simulink model "dig_int_kurt"  (Simulink 6.2)
settings: Solver=ode45  StartTime=0.0  StopTime=1  RelTol=1e-3
undefined symbols (not defined in the file): bit_rev, iBOB, pfb_coeff_gen_calc
libraries: xbsIndex_r3 x1084, casper_library x95, xps_library x32
(part 2 of 8)

== system dig_int_kurt/cram1 ==
  In1 : Inport  Port=1  LatchInput=off
  In2 : Inport  Port=2  LatchInput=off
  In3 : Inport  Port=3  LatchInput=off
  In4 : Inport  Port=4  LatchInput=off
  In5 : Inport  Port=5  LatchInput=off
  In6 : Inport  Port=6  LatchInput=off
  Concat : S-Function  AncestorBlock=xbsIndex_r3/Concat  FunctionName=xlconcat  Parameters=sfcn_mwsv__  mask(Xilinx Bus Concatenator){num_inputs=6, explicit_period=off, period=1, dbl_ovrd=off}
      mask prompts: num_inputs "Number of Inputs"; explicit_period "Use Explicit Sample Period"; period "Sample Period  (use -1 to inherit first known input period)"; dbl_ovrd "Override with Doubles"
      mask help: Concatenates two or more inputs. Inputs must be unsigned with binary point at zero.
      mask init:
      | [designRoot, family, part, speed, package, simulinkPeriod, sysclkPeriod, dbl_ovrd, trimVbit] = xlSysgenSettings(gcb,1,1);
      | [bg,fg] = xlcmap('XBlock',dbl_ovrd);
      | iPos = get_param(gcb,'Position');
      | iWidth=iPos(3)-iPos(1); iHeight=iPos(4)-iPos(2);
      | iCx=iWidth/2;
      | iCy=iHeight/2;
      | [logoX, logoY] = xlogo(iPos);
      | 
      | 
      | 
      | 
      | % one time added for param list
      | numInputs = num_inputs + 1;
      | precision0 = 1;
      | latency = 0;
      | dblOvrd = dbl_ovrd;
      | explicitClk = explicit_period;
      | 
      | 
      | % just pass everything to s-function
      | sfcn_mwsv__ = get_param(gcb, 'MaskWSVariables');
      mask Help: eval('xlWeb(xlhtmldoclink(''Concat''))');
      mask StyleString: popup(2|3|4|5|6|7|8|9|10|11|12|13|14|15|16),checkbox,edit,checkbox
      mask CallbackString: |xlMagicCallback||
      mask Display:
      | patch([0 iWidth iWidth 0],[0 0 iHeight iHeight] , bg);
      | patch(logoX,logoY, fg);
      | port_label('input',1,'hi');
      | port_label('input',num_inputs+1,'lo');
      | port_label('output',1,'cat');
      | ;plot([0 0 iWidth iWidth 0], [0 iHeight iHeight 0 0]);
  Reinterp{1..6} (6 alike) : xbsIndex_r3/Reinterpret  force_arith_type=on  arith_type=Unsigned  force_bin_pt=on  bin_pt=0  force_valid=on
  Out : Outport
  wires:
  Concat/1 -> Out/1
  In1/1 -> Reinterp1/1
  Reinterp1/1 -> Concat/1
  In2/1 -> Reinterp2/1
  Reinterp2/1 -> Concat/2
  In3/1 -> Reinterp3/1
  Reinterp3/1 -> Concat/3
  In4/1 -> Reinterp4/1
  Reinterp4/1 -> Concat/4
  In5/1 -> Reinterp5/1
  Reinterp5/1 -> Concat/5
  In6/1 -> Reinterp6/1
  Reinterp6/1 -> Concat/6

== system dig_int_kurt/cram_crossterms ==
  In1 : Inport  Port=1  LatchInput=off
  In2 : Inport  Port=2  LatchInput=off
  Concat : S-Function  AncestorBlock=xbsIndex_r3/Concat  FunctionName=xlconcat  Parameters=sfcn_mwsv__  mask(Xilinx Bus Concatenator){num_inputs=2, explicit_period=off, period=1, dbl_ovrd=off}
      mask prompts: num_inputs "Number of Inputs"; explicit_period "Use Explicit Sample Period"; period "Sample Period  (use -1 to inherit first known input period)"; dbl_ovrd "Override with Doubles"
      mask help: Concatenates two or more inputs. Inputs must be unsigned with binary point at zero.
      mask init: same as dig_int_kurt/cram1/Concat
      mask Help: eval('xlWeb(xlhtmldoclink(''Concat''))');
      mask StyleString: popup(2|3|4|5|6|7|8|9|10|11|12|13|14|15|16),checkbox,edit,checkbox
      mask CallbackString: |xlMagicCallback||
      mask Display:
      | patch([0 iWidth iWidth 0],[0 0 iHeight iHeight] , bg);
      | patch(logoX,logoY, fg);
      | port_label('input',1,'hi');
      | port_label('input',num_inputs+1,'lo');
      | port_label('output',1,'cat');
      | ;plot([0 0 iWidth iWidth 0], [0 iHeight iHeight 0 0]);
  Reinterp1 : xbsIndex_r3/Reinterpret  force_arith_type=on  arith_type=Unsigned  force_bin_pt=on  bin_pt=0  force_valid=on
  Reinterp2 : xbsIndex_r3/Reinterpret  force_arith_type=on  arith_type=Unsigned  force_bin_pt=on  bin_pt=0  force_valid=on
  Out : Outport
  wires:
  Concat/1 -> Out/1
  In1/1 -> Reinterp1/1
  Reinterp1/1 -> Concat/1
  In2/1 -> Reinterp2/1
  Reinterp2/1 -> Concat/2

== system dig_int_kurt/cram_kurt ==
  In1 : Inport  Port=1  LatchInput=off
  In2 : Inport  Port=2  LatchInput=off
  Concat : S-Function  AncestorBlock=xbsIndex_r3/Concat  FunctionName=xlconcat  Parameters=sfcn_mwsv__  mask(Xilinx Bus Concatenator){num_inputs=2, explicit_period=off, period=1, dbl_ovrd=off}
      mask prompts: num_inputs "Number of Inputs"; explicit_period "Use Explicit Sample Period"; period "Sample Period  (use -1 to inherit first known input period)"; dbl_ovrd "Override with Doubles"
      mask help: Concatenates two or more inputs. Inputs must be unsigned with binary point at zero.
      mask init: same as dig_int_kurt/cram1/Concat
      mask Help: eval('xlWeb(xlhtmldoclink(''Concat''))');
      mask StyleString: popup(2|3|4|5|6|7|8|9|10|11|12|13|14|15|16),checkbox,edit,checkbox
      mask CallbackString: |xlMagicCallback||
      mask Display:
      | patch([0 iWidth iWidth 0],[0 0 iHeight iHeight] , bg);
      | patch(logoX,logoY, fg);
      | port_label('input',1,'hi');
      | port_label('input',num_inputs+1,'lo');
      | port_label('output',1,'cat');
      | ;plot([0 0 iWidth iWidth 0], [0 iHeight iHeight 0 0]);
  Reinterp1 : xbsIndex_r3/Reinterpret  force_arith_type=on  arith_type=Unsigned  force_bin_pt=on  bin_pt=0  force_valid=on
  Reinterp2 : xbsIndex_r3/Reinterpret  force_arith_type=on  arith_type=Unsigned  force_bin_pt=on  bin_pt=0  force_valid=on
  Out : Outport
  wires:
  Reinterp2/1 -> Concat/2
  In2/1 -> Reinterp2/1
  Reinterp1/1 -> Concat/1
  In1/1 -> Reinterp1/1
  Concat/1 -> Out/1

== system dig_int_kurt/cram_powers ==
  In1 : Inport  Port=1  LatchInput=off
  In2 : Inport  Port=2  LatchInput=off
  Concat : S-Function  AncestorBlock=xbsIndex_r3/Concat  FunctionName=xlconcat  Parameters=sfcn_mwsv__  mask(Xilinx Bus Concatenator){num_inputs=2, explicit_period=off, period=1, dbl_ovrd=off}
      mask prompts: num_inputs "Number of Inputs"; explicit_period "Use Explicit Sample Period"; period "Sample Period  (use -1 to inherit first known input period)"; dbl_ovrd "Override with Doubles"
      mask help: Concatenates two or more inputs. Inputs must be unsigned with binary point at zero.
      mask init: same as dig_int_kurt/cram1/Concat
      mask Help: eval('xlWeb(xlhtmldoclink(''Concat''))');
      mask StyleString: popup(2|3|4|5|6|7|8|9|10|11|12|13|14|15|16),checkbox,edit,checkbox
      mask CallbackString: |xlMagicCallback||
      mask Display:
      | patch([0 iWidth iWidth 0],[0 0 iHeight iHeight] , bg);
      | patch(logoX,logoY, fg);
      | port_label('input',1,'hi');
      | port_label('input',num_inputs+1,'lo');
      | port_label('output',1,'cat');
      | ;plot([0 0 iWidth iWidth 0], [0 iHeight iHeight 0 0]);
  Reinterp1 : xbsIndex_r3/Reinterpret  force_arith_type=on  arith_type=Unsigned  force_bin_pt=on  bin_pt=0  force_valid=on
  Reinterp2 : xbsIndex_r3/Reinterpret  force_arith_type=on  arith_type=Unsigned  force_bin_pt=on  bin_pt=0  force_valid=on
  Out : Outport
  wires:
  Concat/1 -> Out/1
  In1/1 -> Reinterp1/1
  Reinterp1/1 -> Concat/1
  In2/1 -> Reinterp2/1
  Reinterp2/1 -> Concat/2

== system dig_int_kurt/fft ==
  sync : Inport  Port=1  LatchInput=off
  shift : Inport  Port=2  LatchInput=off
  pol0 : Inport  Port=3  LatchInput=off
  pol1 : Inport  Port=4  LatchInput=off
  fft_biplex0 : Subsystem  AncestorBlock=casper_library/FFTs/fft_biplex  mask(fft_biplex){FFTSize=10, BitWidth=18, quantization=Truncate, overflow=Wrap, add_latency=3, mult_latency=4, bram_latency=3}
      mask prompts: FFTSize "Size of FFT: (2^? pnts)"; BitWidth "Bitwidth: (Max Efficiency at 18 bits)"; quantization "Quantization Behavior"; overflow "Overflow Behavior"; add_latency "Add Latency"; mult_latency "Mult Latency"; bram_latency "BRAM Latency"
      mask init:
      | fft_biplex_init(gcb,...
      |     'FFTSize', FFTSize,...
      |     'BitWidth', BitWidth,...
      |     'quantization', quantization,...
      |     'overflow', overflow,...
      |     'add_latency', add_latency,...
      |     'mult_latency', mult_latency,...
      |     'bram_latency', bram_latency);
      settings: AttributesFormatString=FFTSize=10, BitWidth=18
      mask StyleString: edit,edit,popup(Truncate|Round  (unbiased: +/- Inf)|Round  (unbiased: Even Values)),popup(Wrap|Saturate|Error),edit,edit,edit
  sync_out : Outport
  out0 : Outport  Port=2
  out1 : Outport  Port=3
  wires:
  pol0/1 -> fft_biplex0/1(pol1)
  pol1/1 -> fft_biplex0/2(pol2)
  shift/1 -> fft_biplex0/4(shift)
  sync/1 -> fft_biplex0/3(sync)
  fft_biplex0/1(pol1_out) -> out0/1
  fft_biplex0/2(pol2_out) -> out1/1
  fft_biplex0/4(sync_out) -> sync_out/1

== system dig_int_kurt/pfb_fir ==
  sync : Inport  Port=1  LatchInput=off
  pol1_in1 : Inport  Port=2  LatchInput=off
  pol2_in1 : Inport  Port=3  LatchInput=off
  pol1_in1_first_tap : Subsystem  AncestorBlock=casper_library/PFBs/first_tap  mask(first_tap){nput=0, PFBSize=10, CoeffBitWidth=8, TotalTaps=4, BitWidthIn=8, CoeffDistMem=1, WindowType=hamming, mult_latency=3, bram_latency=3, n_inputs=0, fwidth=1}
      mask prompts: nput "This is input number:"; PFBSize "Size of PFB: (2^? pnts)"; CoeffBitWidth "Bitwidth of Coefficients:"; TotalTaps "Total Number of Taps:"; BitWidthIn "Input Bitwidth:"; CoeffDistMem "Implement Coeff Gen in Distributed Memory:"; WindowType "Windowing Function:"; mult_latency "Mult Latency"; bram_latency "BRAM Latency"; n_inputs "Number of Simultaneous Inputs: (2^?)"; fwidth "Bit Width (normal=1)"
      mask init:
      | first_tap_init(gcb,...
      |     'nput', nput,...
      |     'PFBSize', PFBSize,...
      |     'CoeffBitWidth', CoeffBitWidth,...
      |     'TotalTaps', TotalTaps,...
      |     'BitWidthIn', BitWidthIn,...
      |     'CoeffDistMem', CoeffDistMem,...
      |     'WindowType', WindowType,...
      |     'mult_latency', mult_latency,...
      |     'bram_latency', bram_latency,...
      |     'n_inputs', n_inputs,...
      |     'fwidth', fwidth);
      settings: AttributesFormatString=input=0, taps=4
      mask StyleString: edit,edit,edit,edit,edit,edit,popup(bartlett|barthannwin|blackman|blackmanharris|bohamwin|chebwin|flattopwin|gausswin|hamming|hann|kaiser|nuttallwin|parzenwin|rectwin|tukeywin|triang),edit,edit,edit,edit
  pol1_in1_last_tap : Subsystem  AncestorBlock=casper_library/PFBs/last_tap  mask(last_tap){TotalTaps=4, BitWidthIn=8, BitWidthOut=18, CoeffBitWidth=8, add_latency=2, mult_latency=3, quantization=Truncate}
      mask prompts: TotalTaps "Total Number of Taps:"; BitWidthIn "Input Bitwidth:"; BitWidthOut "Output Bitwidth:"; CoeffBitWidth "Coeff Bitwidth:"; add_latency "Add Latency"; mult_latency "Mult Latency"; quantization "Quantization Behavior"
      mask init:
      | last_tap_init(gcb,...
      |     'TotalTaps', TotalTaps,...
      |     'BitWidthIn', BitWidthIn,...
      |     'BitWidthOut', BitWidthOut,...
      |     'CoeffBitWidth', CoeffBitWidth,...
      |     'add_latency', add_latency,...
      |     'mult_latency', mult_latency,...
      |     'quantization', quantization);
      settings: AttributesFormatString=taps=4
      mask StyleString: edit,edit,edit,edit,edit,edit,popup(Truncate|Round  (unbiased: +/- Inf)|Round  (unbiased: Even Values))
  pol1_in1_tap2 : casper_library/PFBs/tap
      link override delay/delay_bram/Constant2: equ=P=C
      link override sync_delay/Constant: equ=P=C
      link override sync_delay/Constant1: equ=P=C
      link override sync_delay/Constant2: equ=P=C
      link override sync_delay/Constant3: equ=P=C
  pol1_in1_tap3 : casper_library/PFBs/tap
      link override delay/delay_bram/Constant2: equ=P=C
      link override sync_delay/Constant: equ=P=C
      link override sync_delay/Constant1: equ=P=C
      link override sync_delay/Constant2: equ=P=C
      link override sync_delay/Constant3: equ=P=C
  pol2_in1_first_tap : Subsystem  AncestorBlock=casper_library/PFBs/first_tap  mask(first_tap){nput=0, PFBSize=10, CoeffBitWidth=8, TotalTaps=4, BitWidthIn=8, CoeffDistMem=1, WindowType=hamming, mult_latency=3, bram_latency=3, n_inputs=0, fwidth=1}
      mask prompts: nput "This is input number:"; PFBSize "Size of PFB: (2^? pnts)"; CoeffBitWidth "Bitwidth of Coefficients:"; TotalTaps "Total Number of Taps:"; BitWidthIn "Input Bitwidth:"; CoeffDistMem "Implement Coeff Gen in Distributed Memory:"; WindowType "Windowing Function:"; mult_latency "Mult Latency"; bram_latency "BRAM Latency"; n_inputs "Number of Simultaneous Inputs: (2^?)"; fwidth "Bit Width (normal=1)"
      mask init: same as dig_int_kurt/pfb_fir/pol1_in1_first_tap
      settings: AttributesFormatString=input=0, taps=4
      mask StyleString: edit,edit,edit,edit,edit,edit,popup(bartlett|barthannwin|blackman|blackmanharris|bohamwin|chebwin|flattopwin|gausswin|hamming|hann|kaiser|nuttallwin|parzenwin|rectwin|tukeywin|triang),edit,edit,edit,edit
  pol2_in1_last_tap : Subsystem  AncestorBlock=casper_library/PFBs/last_tap  mask(last_tap){TotalTaps=4, BitWidthIn=8, BitWidthOut=18, CoeffBitWidth=8, add_latency=2, mult_latency=3, quantization=Truncate}
      mask prompts: TotalTaps "Total Number of Taps:"; BitWidthIn "Input Bitwidth:"; BitWidthOut "Output Bitwidth:"; CoeffBitWidth "Coeff Bitwidth:"; add_latency "Add Latency"; mult_latency "Mult Latency"; quantization "Quantization Behavior"
      mask init: same as dig_int_kurt/pfb_fir/pol1_in1_last_tap
      settings: AttributesFormatString=taps=4
      mask StyleString: edit,edit,edit,edit,edit,edit,popup(Truncate|Round  (unbiased: +/- Inf)|Round  (unbiased: Even Values))
  pol2_in1_tap2 : casper_library/PFBs/tap
      link override delay/delay_bram/Constant2: equ=P=C
      link override sync_delay/Constant: equ=P=C
      link override sync_delay/Constant1: equ=P=C
      link override sync_delay/Constant2: equ=P=C
      link override sync_delay/Constant3: equ=P=C
  pol2_in1_tap3 : casper_library/PFBs/tap
      link override delay/delay_bram/Constant2: equ=P=C
      link override sync_delay/Constant: equ=P=C
      link override sync_delay/Constant1: equ=P=C
      link override sync_delay/Constant2: equ=P=C
      link override sync_delay/Constant3: equ=P=C
  sync_out : Outport
  pol1_out1 : Outport  Port=2
  pol2_out1 : Outport  Port=3
  wires:
  pol1_in1/1 -> pol1_in1_first_tap/1(din)
  sync/1 -> pol1_in1_first_tap/2(sync), pol2_in1_first_tap/2(sync)
  pol1_in1_first_tap/1(dout) -> pol1_in1_tap2/1
  pol1_in1_first_tap/2(sync_out) -> pol1_in1_tap2/2
  pol1_in1_first_tap/3(coeff_out) -> pol1_in1_tap2/3
  pol1_in1_first_tap/4(taps_out) -> pol1_in1_tap2/4
  pol1_in1_tap2/1 -> pol1_in1_tap3/1
  pol1_in1_tap2/2 -> pol1_in1_tap3/2
  pol1_in1_tap2/3 -> pol1_in1_tap3/3
  pol1_in1_tap2/4 -> pol1_in1_tap3/4
  pol1_in1_tap3/1 -> pol1_in1_last_tap/1(din)
  pol1_in1_tap3/2 -> pol1_in1_last_tap/2(sync)
  pol1_in1_tap3/3 -> pol1_in1_last_tap/3(coeff)
  pol1_in1_tap3/4 -> pol1_in1_last_tap/4(taps)
  pol1_in1_last_tap/1(dout) -> pol1_out1/1
  pol1_in1_last_tap/2(sync_out) -> sync_out/1
  pol2_in1/1 -> pol2_in1_first_tap/1(din)
  pol2_in1_first_tap/1(dout) -> pol2_in1_tap2/1
  pol2_in1_first_tap/2(sync_out) -> pol2_in1_tap2/2
  pol2_in1_first_tap/3(coeff_out) -> pol2_in1_tap2/3
  pol2_in1_first_tap/4(taps_out) -> pol2_in1_tap2/4
  pol2_in1_tap2/1 -> pol2_in1_tap3/1
  pol2_in1_tap2/2 -> pol2_in1_tap3/2
  pol2_in1_tap2/3 -> pol2_in1_tap3/3
  pol2_in1_tap2/4 -> pol2_in1_tap3/4
  pol2_in1_tap3/1 -> pol2_in1_last_tap/1(din)
  pol2_in1_tap3/2 -> pol2_in1_last_tap/2(sync)
  pol2_in1_tap3/3 -> pol2_in1_last_tap/3(coeff)
  pol2_in1_tap3/4 -> pol2_in1_last_tap/4(taps)
  pol2_in1_last_tap/1(dout) -> pol2_out1/1

== system dig_int_kurt/pol1_kurt1 ==
  note: Input unsigned 24-bits, b.p. at 23
  note: Output unsigned 24-bits, b.p. at 23
  note: Unsigned, 18-bits, b.p. at 12
  coeff : Inport  Orientation=down  Port=1  LatchInput=off
  data_in : Inport  Port=2  LatchInput=off
  Convert : xbsIndex_r3/Convert  arith_type=Unsigned  n_bits=24  bin_pt=23  quantization=Truncate  overflow=Wrap  latency=1  explicit_period=off  period=1  dbl_ovrd=off  show_param=off  inserted_by_tool=off  pipeline=off
      settings: xl_area=[0, 0, 0, 0, 0, 0, 0]
  mult_coeff_fft_real : xbsIndex_r3/Mult  precision=Full  arith_type="Signed  (2's comp)"  n_bits=24  bin_pt=23  quantization=Truncate  overflow=Wrap  latency=5  explicit_period=off  period=1  en=off  dbl_ovrd=off  show_param=on  mult_type=Parallel  oversample=2  use_embedded=on  pipeline=on  use_rpm=on  placement_style=Rectangular Shape  gen_core=off
      settings: xl_area=[0, 0, 0, 0, 0, 0, 0]
  data_out : Outport
  wires:
  Convert/1 -> data_out/1
  data_in/1 -> mult_coeff_fft_real/2
  coeff/1 -> mult_coeff_fft_real/1
  mult_coeff_fft_real/1 -> Convert/1

== system dig_int_kurt/pol2_kurt1 ==
  note: Unsigned, 18-bits, b.p. at 12
  note: Output unsigned 24-bits, b.p. at 23
  note: Input unsigned 24-bits, b.p. at 23
  coeff : Inport  Orientation=down  Port=1  LatchInput=off
  data_in : Inport  Port=2  LatchInput=off
  Convert : xbsIndex_r3/Convert  arith_type=Unsigned  n_bits=24  bin_pt=23  quantization=Truncate  overflow=Wrap  latency=1  explicit_period=off  period=1  dbl_ovrd=off  show_param=off  inserted_by_tool=off  pipeline=off
      settings: xl_area=[0, 0, 0, 0, 0, 0, 0]
  mult_coeff_fft_real : xbsIndex_r3/Mult  precision=Full  arith_type="Signed  (2's comp)"  n_bits=24  bin_pt=23  quantization=Truncate  overflow=Wrap  latency=5  explicit_period=off  period=1  en=off  dbl_ovrd=off  show_param=on  mult_type=Parallel  oversample=2  use_embedded=on  pipeline=on  use_rpm=on  placement_style=Rectangular Shape  gen_core=off
      settings: xl_area=[0, 0, 0, 0, 0, 0, 0]
  data_out : Outport
  wires:
  Convert/1 -> data_out/1
  mult_coeff_fft_real/1 -> Convert/1
  coeff/1 -> mult_coeff_fft_real/1
  data_in/1 -> mult_coeff_fft_real/2

== system dig_int_kurt/signed_bitselect_2 ==
  note: Selects the bits 16-22 (inclusive) and a sign bit.
  note: Selects the bits 8-14 (inclusive) and a sign bit.
  note: Selects the bits 0-6 (inclusive) and a sign bit.
  note: Selects the bits 24-30 (inclusive) and a sign bit.
  bitselect : Inport  Port=1  LatchInput=off
  data_in : Inport  Port=2  LatchInput=off
  Convert{,1..3} (4 alike) : xbsIndex_r3/Convert  arith_type="Signed  (2's comp)"  n_bits=8  bin_pt=7  quantization="Round  (unbiased: +/- Inf)"  overflow=Saturate  latency=1  explicit_period=off  period=1  dbl_ovrd=off  show_param=off  inserted_by_tool=off  pipeline=off
      settings: xl_area=[0, 0, 0, 0, 0, 0, 0]
  Mux : xbsIndex_r3/Mux  inputs=4  precision=Full  arith_type="Signed  (2's comp)"  n_bits=8  bin_pt=2  quantization=Truncate  overflow=Wrap  latency=0  explicit_period=off  period=1  en=off  dbl_ovrd=off  show_param=off  mux_type=off  use_rpm=off  gen_core=off
      settings: xl_area=[0, 0, 0, 0, 0, 0, 0]
  Reinterpret{,1..3} (4 alike) : xbsIndex_r3/Reinterpret  force_arith_type=on  arith_type=Unsigned  force_bin_pt=on  bin_pt=0  force_valid=on
  Scale : xbsIndex_r3/Scale  scale_factor=-8  explicit_period=off  period=1  dbl_ovrd=off
  Scale1 : xbsIndex_r3/Scale  scale_factor=8  explicit_period=off  period=1  dbl_ovrd=off
  Scale2 : xbsIndex_r3/Scale  scale_factor=16  explicit_period=off  period=1  dbl_ovrd=off
  data_out : Outport
  wires:
  data_in/1 -> Scale/1, Convert1/1, Scale1/1, Scale2/1
  Convert/1 -> Reinterpret/1
  Scale/1 -> Convert/1
  Mux/1 -> data_out/1
  Convert1/1 -> Reinterpret1/1
  Convert2/1 -> Reinterpret2/1
  Scale1/1 -> Convert2/1
  Reinterpret/1 -> Mux/2
  Reinterpret1/1 -> Mux/3
  Reinterpret2/1 -> Mux/4
  Convert3/1 -> Reinterpret3/1
  Scale2/1 -> Convert3/1
  Reinterpret3/1 -> Mux/5
  bitselect/1 -> Mux/1

== system dig_int_kurt/signed_bitselect_3 ==
  note: Selects the bits 24-30 (inclusive) and a sign bit.
  note: Selects the bits 0-6 (inclusive) and a sign bit.
  note: Selects the bits 8-14 (inclusive) and a sign bit.
  note: Selects the bits 16-22 (inclusive) and a sign bit.
  bitselect : Inport  Port=1  LatchInput=off
  data_in : Inport  Port=2  LatchInput=off
  Convert{,1..3} (4 alike) : xbsIndex_r3/Convert  arith_type="Signed  (2's comp)"  n_bits=8  bin_pt=7  quantization="Round  (unbiased: +/- Inf)"  overflow=Saturate  latency=1  explicit_period=off  period=1  dbl_ovrd=off  show_param=off  inserted_by_tool=off  pipeline=off
      settings: xl_area=[0, 0, 0, 0, 0, 0, 0]
  Mux : xbsIndex_r3/Mux  inputs=4  precision=Full  arith_type="Signed  (2's comp)"  n_bits=8  bin_pt=2  quantization=Truncate  overflow=Wrap  latency=0  explicit_period=off  period=1  en=off  dbl_ovrd=off  show_param=off  mux_type=off  use_rpm=off  gen_core=off
      settings: xl_area=[0, 0, 0, 0, 0, 0, 0]
  Reinterpret{,1..3} (4 alike) : xbsIndex_r3/Reinterpret  force_arith_type=on  arith_type=Unsigned  force_bin_pt=on  bin_pt=0  force_valid=on
  Scale : xbsIndex_r3/Scale  scale_factor=-8  explicit_period=off  period=1  dbl_ovrd=off
  Scale1 : xbsIndex_r3/Scale  scale_factor=8  explicit_period=off  period=1  dbl_ovrd=off
  Scale2 : xbsIndex_r3/Scale  scale_factor=16  explicit_period=off  period=1  dbl_ovrd=off
  data_out : Outport
  wires:
  bitselect/1 -> Mux/1
  Reinterpret3/1 -> Mux/5
  Scale2/1 -> Convert3/1
  Convert3/1 -> Reinterpret3/1
  Reinterpret2/1 -> Mux/4
  Reinterpret1/1 -> Mux/3
  Reinterpret/1 -> Mux/2
  Scale1/1 -> Convert2/1
  Convert2/1 -> Reinterpret2/1
  Convert1/1 -> Reinterpret1/1
  Mux/1 -> data_out/1
  Scale/1 -> Convert/1
  Convert/1 -> Reinterpret/1
  data_in/1 -> Scale2/1, Scale1/1, Convert1/1, Scale/1

== system dig_int_kurt/signed_scale2 ==
  note: Input signed 24-bits, b.p. at 23
  note: Output signed 24-bits, b.p. at 23
  note: Unsigned, 18-bits, b.p. at 12
  coeff : Inport  Orientation=down  Port=1  LatchInput=off
  data_in : Inport  Port=2  LatchInput=off
  Convert : xbsIndex_r3/Convert  arith_type="Signed  (2's comp)"  n_bits=24  bin_pt=23  quantization=Truncate  overflow=Wrap  latency=1  explicit_period=off  period=1  dbl_ovrd=off  show_param=off  inserted_by_tool=off  pipeline=off
      settings: xl_area=[0, 0, 0, 0, 0, 0, 0]
  mult_coeff_fft_real : xbsIndex_r3/Mult  precision=Full  arith_type="Signed  (2's comp)"  n_bits=24  bin_pt=23  quantization=Truncate  overflow=Wrap  latency=5  explicit_period=off  period=1  en=off  dbl_ovrd=off  show_param=on  mult_type=Parallel  oversample=2  use_embedded=on  pipeline=on  use_rpm=on  placement_style=Rectangular Shape  gen_core=off
      settings: xl_area=[0, 0, 0, 0, 0, 0, 0]
  data_out : Outport
  wires:
  data_in/1 -> mult_coeff_fft_real/2
  coeff/1 -> mult_coeff_fft_real/1
  mult_coeff_fft_real/1 -> Convert/1
  Convert/1 -> data_out/1

== system dig_int_kurt/signed_scale3 ==
  note: Unsigned, 18-bits, b.p. at 12
  note: Output signed 24-bits, b.p. at 23
  note: Input signed 24-bits, b.p. at 23
  coeff : Inport  Orientation=down  Port=1  LatchInput=off
  data_in : Inport  Port=2  LatchInput=off
  Convert : xbsIndex_r3/Convert  arith_type="Signed  (2's comp)"  n_bits=24  bin_pt=23  quantization=Truncate  overflow=Wrap  latency=1  explicit_period=off  period=1  dbl_ovrd=off  show_param=off  inserted_by_tool=off  pipeline=off
      settings: xl_area=[0, 0, 0, 0, 0, 0, 0]
  mult_coeff_fft_real : xbsIndex_r3/Mult  precision=Full  arith_type="Signed  (2's comp)"  n_bits=24  bin_pt=23  quantization=Truncate  overflow=Wrap  latency=5  explicit_period=off  period=1  en=off  dbl_ovrd=off  show_param=on  mult_type=Parallel  oversample=2  use_embedded=on  pipeline=on  use_rpm=on  placement_style=Rectangular Shape  gen_core=off
      settings: xl_area=[0, 0, 0, 0, 0, 0, 0]
  data_out : Outport
  wires:
  mult_coeff_fft_real/1 -> Convert/1
  coeff/1 -> mult_coeff_fft_real/1
  data_in/1 -> mult_coeff_fft_real/2
  Convert/1 -> data_out/1

== system dig_int_kurt/sync_generator ==
  period : Inport  Port=1  LatchInput=off
  reset : Inport  Port=2  LatchInput=off
  Convert : xbsIndex_r3/Convert  arith_type=Boolean  n_bits=8  bin_pt=6  quantization=Truncate  overflow=Wrap  latency=1  explicit_period=off  period=1  dbl_ovrd=off  show_param=off  inserted_by_tool=off  pipeline=off
      settings: xl_area=[0, 0, 0, 0, 0, 0, 0]
  Counter : xbsIndex_r3/Counter  cnt_type=Free Running  n_bits=32  bin_pt=0  arith_type=Unsigned  start_count=1  cnt_to=Inf  cnt_by_val=1  operation=Up  explicit_period=on  period=1  load_pin=off  rst=on  en=off  dbl_ovrd=off  show_param=off  use_rpm=on  gen_core=off
      settings: xl_area=[0, 0, 0, 0, 0, 0, 0]
  Logical : xbsIndex_r3/Logical  logical_function=OR  inputs=2  precision=Full  arith_type=Unsigned  n_bits=8  bin_pt=2  align_bp=on  latency=0  explicit_period=off  period=1  en=off  dbl_ovrd=off  show_param=off
      settings: xl_area=[0, 0, 0, 0, 0, 0, 0]
  Relational : xbsIndex_r3/Relational  mode=a>=b  latency=1  explicit_period=off  period=1  en=off  dbl_ovrd=off  show_param=off
      settings: xl_area=[0, 0, 0, 0, 0, 0, 0]
  cns : xbsIndex_r3/Constant  const=4  equ=P=C  arith_type=Unsigned  n_bits=3  bin_pt=0  opselect=C  inp2=PCIN>>17  opr=+  inp1=P  carry=CIN  iostate=0  explicit_period=off  period=1  dbl_ovrd=off
  period_sub : xbsIndex_r3/AddSub  mode=Subtraction  precision=User Defined  arith_type=Unsigned  n_bits=32  bin_pt=0  quantization=Truncate  overflow=Wrap  latency=0  explicit_period=off  period=1  use_carryin=off  use_carryout=off  en=off  dbl_ovrd=off  show_param=off  use_core=on  pipeline=off  use_rpm=on  gen_core=off
      settings: xl_area=[0, 0, 0, 0, 0, 0, 0]
  posedge : casper_library/Misc/posedge  Tag=Rising Edge Detector
  sync : Outport
  wires:
  Counter/1 -> Relational/1
  Relational/1 -> Convert/1
  Convert/1 -> Logical/2
  Logical/1 -> Counter/1, posedge/1
  reset/1 -> Logical/1
  period/1 -> period_sub/1
  period_sub/1 -> Relational/2
  cns/1 -> period_sub/2
  posedge/1 -> sync/1

== system dig_int_kurt/uncram_crossterms ==
  In : Inport  Port=1  LatchInput=off
  Reinterp1 : xbsIndex_r3/Reinterpret  force_arith_type=on  arith_type="Signed  (2's comp)"  force_bin_pt=on  bin_pt=23  force_valid=on
  Reinterp2 : xbsIndex_r3/Reinterpret  force_arith_type=on  arith_type="Signed  (2's comp)"  force_bin_pt=on  bin_pt=23  force_valid=on
  Slice1 : xbsIndex_r3/Slice  mode=Upper Bit Location + Width  nbits=32  bit1=0  base1=MSB of Input  bit0=0  base0=LSB of Input  boolean_output=off  explicit_period=off  period=1  dbl_ovrd=off
  Slice2 : xbsIndex_r3/Slice  mode=Upper Bit Location + Width  nbits=32  bit1=-32  base1=MSB of Input  bit0=0  base0=LSB of Input  boolean_output=off  explicit_period=off  period=1  dbl_ovrd=off
  Out1 : Outport
  Out2 : Outport  Port=2
  wires:
  In/1 -> Slice1/1, Slice2/1
  Slice1/1 -> Reinterp1/1
  Reinterp1/1 -> Out1/1
  Slice2/1 -> Reinterp2/1
  Reinterp2/1 -> Out2/1

== system dig_int_kurt/uncram_powers ==
  In : Inport  Port=1  LatchInput=off
  Reinterp1 : xbsIndex_r3/Reinterpret  force_arith_type=on  arith_type=Unsigned  force_bin_pt=on  bin_pt=23  force_valid=on
  Reinterp2 : xbsIndex_r3/Reinterpret  force_arith_type=on  arith_type=Unsigned  force_bin_pt=on  bin_pt=23  force_valid=on
  Slice1 : xbsIndex_r3/Slice  mode=Upper Bit Location + Width  nbits=32  bit1=0  base1=MSB of Input  bit0=0  base0=LSB of Input  boolean_output=off  explicit_period=off  period=1  dbl_ovrd=off
  Slice2 : xbsIndex_r3/Slice  mode=Upper Bit Location + Width  nbits=32  bit1=-32  base1=MSB of Input  bit0=0  base0=LSB of Input  boolean_output=off  explicit_period=off  period=1  dbl_ovrd=off
  Out1 : Outport
  Out2 : Outport  Port=2
  wires:
  In/1 -> Slice1/1, Slice2/1
  Slice1/1 -> Reinterp1/1
  Reinterp1/1 -> Out1/1
  Slice2/1 -> Reinterp2/1
  Reinterp2/1 -> Out2/1

== system dig_int_kurt/uncram_powers1 ==
  In : Inport  Port=1  LatchInput=off
  Reinterp1 : xbsIndex_r3/Reinterpret  force_arith_type=on  arith_type=Unsigned  force_bin_pt=on  bin_pt=23  force_valid=on
  Reinterp2 : xbsIndex_r3/Reinterpret  force_arith_type=on  arith_type=Unsigned  force_bin_pt=on  bin_pt=23  force_valid=on
  Slice1 : xbsIndex_r3/Slice  mode=Upper Bit Location + Width  nbits=48  bit1=0  base1=MSB of Input  bit0=0  base0=LSB of Input  boolean_output=off  explicit_period=off  period=1  dbl_ovrd=off
  Slice2 : xbsIndex_r3/Slice  mode=Upper Bit Location + Width  nbits=48  bit1=-48  base1=MSB of Input  bit0=0  base0=LSB of Input  boolean_output=off  explicit_period=off  period=1  dbl_ovrd=off
  Out1 : Outport
  Out2 : Outport  Port=2
  wires:
  In/1 -> Slice1/1, Slice2/1
  Slice1/1 -> Reinterp1/1
  Reinterp1/1 -> Out1/1
  Slice2/1 -> Reinterp2/1
  Reinterp2/1 -> Out2/1

== system dig_int_kurt/unsigned_bitselect_1 ==
  bitselect : Inport  Port=1  LatchInput=off
  data_in : Inport  Port=2  LatchInput=off
  mux_bitselect : xbsIndex_r3/Mux  inputs=4  precision=Full  arith_type="Signed  (2's comp)"  n_bits=8  bin_pt=2  quantization=Truncate  overflow=Wrap  latency=1  explicit_period=off  period=1  en=off  dbl_ovrd=off  show_param=off  mux_type=off  use_rpm=off  gen_core=off
      settings: xl_area=[0, 0, 0, 0, 0, 0, 0]
  reint_bp_0 : xbsIndex_r3/Reinterpret  force_arith_type=on  arith_type=Unsigned  force_bin_pt=on  bin_pt=0  force_valid=on
  slc_bitselect_1 : xbsIndex_r3/Slice  mode=Lower Bit Location + Width  nbits=8  bit1=0  base1=MSB of Input  bit0=0  base0=LSB of Input  boolean_output=off  explicit_period=off  period=1  dbl_ovrd=off
  slc_bitselect_2 : xbsIndex_r3/Slice  mode=Lower Bit Location + Width  nbits=8  bit1=0  base1=MSB of Input  bit0=8  base0=LSB of Input  boolean_output=off  explicit_period=off  period=1  dbl_ovrd=off
  slc_bitselect_3 : xbsIndex_r3/Slice  mode=Lower Bit Location + Width  nbits=8  bit1=0  base1=MSB of Input  bit0=16  base0=LSB of Input  boolean_output=off  explicit_period=off  period=1  dbl_ovrd=off
  slc_bitselect_4 : xbsIndex_r3/Slice  mode=Lower Bit Location + Width  nbits=8  bit1=0  base1=MSB of Input  bit0=24  base0=LSB of Input  boolean_output=off  explicit_period=off  period=1  dbl_ovrd=off
  data_out : Outport
  wires:
  reint_bp_0/1 -> slc_bitselect_1/1, slc_bitselect_2/1, slc_bitselect_3/1, slc_bitselect_4/1
  mux_bitselect/1 -> data_out/1
  bitselect/1 -> mux_bitselect/1
  data_in/1 -> reint_bp_0/1
  slc_bitselect_4/1 -> mux_bitselect/5
  slc_bitselect_3/1 -> mux_bitselect/4
  slc_bitselect_2/1 -> mux_bitselect/3
  slc_bitselect_1/1 -> mux_bitselect/2

== system dig_int_kurt/unsigned_bitselect_2 ==
  bitselect : Inport  Port=1  LatchInput=off
  data_in : Inport  Port=2  LatchInput=off
  mux_bitselect : xbsIndex_r3/Mux  inputs=5  precision=Full  arith_type="Signed  (2's comp)"  n_bits=8  bin_pt=2  quantization=Truncate  overflow=Wrap  latency=1  explicit_period=off  period=1  en=off  dbl_ovrd=off  show_param=off  mux_type=off  use_rpm=off  gen_core=off
      settings: xl_area=[0, 0, 0, 0, 0, 0, 0]
  reint_bp_0 : xbsIndex_r3/Reinterpret  force_arith_type=on  arith_type=Unsigned  force_bin_pt=on  bin_pt=0  force_valid=on
  slc_bitselect_1 : xbsIndex_r3/Slice  mode=Lower Bit Location + Width  nbits=16  bit1=0  base1=MSB of Input  bit0=0  base0=LSB of Input  boolean_output=off  explicit_period=off  period=1  dbl_ovrd=off
  slc_bitselect_2 : xbsIndex_r3/Slice  mode=Lower Bit Location + Width  nbits=16  bit1=0  base1=MSB of Input  bit0=8  base0=LSB of Input  boolean_output=off  explicit_period=off  period=1  dbl_ovrd=off
  slc_bitselect_3 : xbsIndex_r3/Slice  mode=Lower Bit Location + Width  nbits=16  bit1=0  base1=MSB of Input  bit0=16  base0=LSB of Input  boolean_output=off  explicit_period=off  period=1  dbl_ovrd=off
  slc_bitselect_4 : xbsIndex_r3/Slice  mode=Lower Bit Location + Width  nbits=16  bit1=0  base1=MSB of Input  bit0=24  base0=LSB of Input  boolean_output=off  explicit_period=off  period=1  dbl_ovrd=off
  slc_bitselect_5 : xbsIndex_r3/Slice  mode=Lower Bit Location + Width  nbits=16  bit1=0  base1=MSB of Input  bit0=32  base0=LSB of Input  boolean_output=off  explicit_period=off  period=1  dbl_ovrd=off
  data_out : Outport
  wires:
  reint_bp_0/1 -> slc_bitselect_1/1, slc_bitselect_2/1, slc_bitselect_3/1, slc_bitselect_4/1, slc_bitselect_5/1
  mux_bitselect/1 -> data_out/1
  bitselect/1 -> mux_bitselect/1
  data_in/1 -> reint_bp_0/1
  slc_bitselect_4/1 -> mux_bitselect/5
  slc_bitselect_3/1 -> mux_bitselect/4
  slc_bitselect_2/1 -> mux_bitselect/3
  slc_bitselect_1/1 -> mux_bitselect/2
  slc_bitselect_5/1 -> mux_bitselect/6

== system dig_int_kurt/unsigned_bitselect_3 ==
  bitselect : Inport  Port=1  LatchInput=off
  data_in : Inport  Port=2  LatchInput=off
  mux_bitselect : xbsIndex_r3/Mux  inputs=5  precision=Full  arith_type="Signed  (2's comp)"  n_bits=8  bin_pt=2  quantization=Truncate  overflow=Wrap  latency=1  explicit_period=off  period=1  en=off  dbl_ovrd=off  show_param=off  mux_type=off  use_rpm=off  gen_core=off
      settings: xl_area=[0, 0, 0, 0, 0, 0, 0]
  reint_bp_0 : xbsIndex_r3/Reinterpret  force_arith_type=on  arith_type=Unsigned  force_bin_pt=on  bin_pt=0  force_valid=on
  slc_bitselect_1 : xbsIndex_r3/Slice  mode=Lower Bit Location + Width  nbits=16  bit1=0  base1=MSB of Input  bit0=0  base0=LSB of Input  boolean_output=off  explicit_period=off  period=1  dbl_ovrd=off
  slc_bitselect_2 : xbsIndex_r3/Slice  mode=Lower Bit Location + Width  nbits=16  bit1=0  base1=MSB of Input  bit0=8  base0=LSB of Input  boolean_output=off  explicit_period=off  period=1  dbl_ovrd=off
  slc_bitselect_3 : xbsIndex_r3/Slice  mode=Lower Bit Location + Width  nbits=16  bit1=0  base1=MSB of Input  bit0=16  base0=LSB of Input  boolean_output=off  explicit_period=off  period=1  dbl_ovrd=off
  slc_bitselect_4 : xbsIndex_r3/Slice  mode=Lower Bit Location + Width  nbits=16  bit1=0  base1=MSB of Input  bit0=24  base0=LSB of Input  boolean_output=off  explicit_period=off  period=1  dbl_ovrd=off
  slc_bitselect_5 : xbsIndex_r3/Slice  mode=Lower Bit Location + Width  nbits=16  bit1=0  base1=MSB of Input  bit0=32  base0=LSB of Input  boolean_output=off  explicit_period=off  period=1  dbl_ovrd=off
  data_out : Outport
  wires:
  slc_bitselect_1/1 -> mux_bitselect/2
  slc_bitselect_2/1 -> mux_bitselect/3
  slc_bitselect_3/1 -> mux_bitselect/4
  slc_bitselect_4/1 -> mux_bitselect/5
  data_in/1 -> reint_bp_0/1
  bitselect/1 -> mux_bitselect/1
  mux_bitselect/1 -> data_out/1
  reint_bp_0/1 -> slc_bitselect_3/1, slc_bitselect_4/1, slc_bitselect_5/1, slc_bitselect_2/1, slc_bitselect_1/1
  slc_bitselect_5/1 -> mux_bitselect/6

== system dig_int_kurt/unsigned_bitselect_4 ==
  bitselect : Inport  Port=1  LatchInput=off
  data_in : Inport  Port=2  LatchInput=off
  mux_bitselect : xbsIndex_r3/Mux  inputs=4  precision=Full  arith_type="Signed  (2's comp)"  n_bits=8  bin_pt=2  quantization=Truncate  overflow=Wrap  latency=1  explicit_period=off  period=1  en=off  dbl_ovrd=off  show_param=off  mux_type=off  use_rpm=off  gen_core=off
      settings: xl_area=[0, 0, 0, 0, 0, 0, 0]
  reint_bp_0 : xbsIndex_r3/Reinterpret  force_arith_type=on  arith_type=Unsigned  force_bin_pt=on  bin_pt=0  force_valid=on
  slc_bitselect_1 : xbsIndex_r3/Slice  mode=Lower Bit Location + Width  nbits=8  bit1=0  base1=MSB of Input  bit0=0  base0=LSB of Input  boolean_output=off  explicit_period=off  period=1  dbl_ovrd=off
  slc_bitselect_2 : xbsIndex_r3/Slice  mode=Lower Bit Location + Width  nbits=8  bit1=0  base1=MSB of Input  bit0=8  base0=LSB of Input  boolean_output=off  explicit_period=off  period=1  dbl_ovrd=off
  slc_bitselect_3 : xbsIndex_r3/Slice  mode=Lower Bit Location + Width  nbits=8  bit1=0  base1=MSB of Input  bit0=16  base0=LSB of Input  boolean_output=off  explicit_period=off  period=1  dbl_ovrd=off
  slc_bitselect_4 : xbsIndex_r3/Slice  mode=Lower Bit Location + Width  nbits=8  bit1=0  base1=MSB of Input  bit0=24  base0=LSB of Input  boolean_output=off  explicit_period=off  period=1  dbl_ovrd=off
  data_out : Outport
  wires:
  slc_bitselect_1/1 -> mux_bitselect/2
  slc_bitselect_2/1 -> mux_bitselect/3
  slc_bitselect_3/1 -> mux_bitselect/4
  slc_bitselect_4/1 -> mux_bitselect/5
  data_in/1 -> reint_bp_0/1
  bitselect/1 -> mux_bitselect/1
  mux_bitselect/1 -> data_out/1
  reint_bp_0/1 -> slc_bitselect_4/1, slc_bitselect_3/1, slc_bitselect_2/1, slc_bitselect_1/1

== system dig_int_kurt/unsigned_scale1 ==
  note: Unsigned, 18-bits, b.p. at 12
  note: Output unsigned 24-bits, b.p. at 23
  note: Input unsigned 24-bits, b.p. at 23
  coeff : Inport  Orientation=down  Port=1  LatchInput=off
  data_in : Inport  Port=2  LatchInput=off
  Convert : xbsIndex_r3/Convert  arith_type=Unsigned  n_bits=24  bin_pt=23  quantization=Truncate  overflow=Wrap  latency=1  explicit_period=off  period=1  dbl_ovrd=off  show_param=off  inserted_by_tool=off  pipeline=off
      settings: xl_area=[0, 0, 0, 0, 0, 0, 0]
  mult_coeff_fft_real : xbsIndex_r3/Mult  precision=Full  arith_type="Signed  (2's comp)"  n_bits=24  bin_pt=23  quantization=Truncate  overflow=Wrap  latency=5  explicit_period=off  period=1  en=off  dbl_ovrd=off  show_param=on  mult_type=Parallel  oversample=2  use_embedded=on  pipeline=on  use_rpm=on  placement_style=Rectangular Shape  gen_core=off
      settings: xl_area=[0, 0, 0, 0, 0, 0, 0]
  data_out : Outport
  wires:
  mult_coeff_fft_real/1 -> Convert/1
  coeff/1 -> mult_coeff_fft_real/1
  data_in/1 -> mult_coeff_fft_real/2
  Convert/1 -> data_out/1

== system dig_int_kurt/unsigned_scale2 ==
  note: Input unsigned 24-bits, b.p. at 23
  note: Output unsigned 24-bits, b.p. at 23
  note: Unsigned, 18-bits, b.p. at 12
  coeff : Inport  Orientation=down  Port=1  LatchInput=off
  data_in : Inport  Port=2  LatchInput=off
  Convert : xbsIndex_r3/Convert  arith_type=Unsigned  n_bits=24  bin_pt=23  quantization=Truncate  overflow=Wrap  latency=1  explicit_period=off  period=1  dbl_ovrd=off  show_param=off  inserted_by_tool=off  pipeline=off
      settings: xl_area=[0, 0, 0, 0, 0, 0, 0]
  mult_coeff_fft_real : xbsIndex_r3/Mult  precision=Full  arith_type="Signed  (2's comp)"  n_bits=24  bin_pt=23  quantization=Truncate  overflow=Wrap  latency=5  explicit_period=off  period=1  en=off  dbl_ovrd=off  show_param=on  mult_type=Parallel  oversample=2  use_embedded=on  pipeline=on  use_rpm=on  placement_style=Rectangular Shape  gen_core=off
      settings: xl_area=[0, 0, 0, 0, 0, 0, 0]
  data_out : Outport
  wires:
  data_in/1 -> mult_coeff_fft_real/2
  coeff/1 -> mult_coeff_fft_real/1
  mult_coeff_fft_real/1 -> Convert/1
  Convert/1 -> data_out/1

== system dig_int_kurt/vacc ==
  note: The slice selects the upper bits of the
      | counter which represent the vector number.
  note: Acc Len is the total number of vectors accumulated minus one
      | Thus acc_len = 0 causes no accumulation, the data is passed through
  note: Valid goes high when dout
      | represents a valid accumulation
  note: ValidDelay should be equal to
      | Add Latency + Mux Latency to align the valid pulse with the output data.
  note: We want to generate a sync pulse that
      | will reset the counter right when the low bits
      | would roll over from veclen-1 to 0 so we need
      | to compare to veclen-2 to take into account
      | the latency in the comparator
  sync : Inport  Port=1  LatchInput=off
  din : Inport  Port=2  LatchInput=off
  acc_len : Inport  Port=3  LatchInput=off
  AND : xbsIndex_r3/Logical  logical_function=AND  inputs=2  precision=Full  arith_type=Unsigned  n_bits=8  bin_pt=2  align_bp=on  latency=0  explicit_period=off  period=1  en=off  dbl_ovrd=off  show_param=off
      settings: xl_area=[0, 0, 0, 0, 0, 0, 0]
  AccEnCompare : xbsIndex_r3/Relational  mode=a!=b  latency=1  explicit_period=off  period=1  en=off  dbl_ovrd=off  show_param=off
      settings: xl_area=[0, 0, 0, 0, 0, 0, 0]
  Counter : xbsIndex_r3/Counter  cnt_type=Free Running  n_bits=18  bin_pt=0  arith_type=Unsigned  start_count=0  cnt_to=Inf  cnt_by_val=1  operation=Up  explicit_period=on  period=1  load_pin=off  rst=on  en=off  dbl_ovrd=off  show_param=off  use_rpm=on  gen_core=off
      settings: xl_area=[0, 0, 0, 0, 0, 0, 0]
  Cram : Subsystem  AncestorBlock=gavrt_library/cram  mask(cram){num_slice=2}
      mask prompts: num_slice "Number of slices"
      mask help: Concatenates inputs together after forcing binary point to zero.
      mask init:
      | cram_init(gcb, ...
      |     'num_slice', num_slice);
  DinDelay : xbsIndex_r3/Delay  latency=2  reg_retiming=on  explicit_period=off  period=1  en=off  accept_only_valid=off  init_zero=on  dbl_ovrd=off  show_param=off
      settings: xl_area=[0, 0, 0, 0, 0, 0, 0]
  OR : xbsIndex_r3/Logical  logical_function=OR  inputs=2  precision=Full  arith_type=Unsigned  n_bits=8  bin_pt=2  align_bp=on  latency=0  explicit_period=off  period=1  en=off  dbl_ovrd=off  show_param=off
      settings: xl_area=[0, 0, 0, 0, 0, 0, 0]
  Slice : xbsIndex_r3/Slice  mode=Upper Bit Location + Width  nbits=8  bit1=0  base1=MSB of Input  bit0=0  base0=LSB of Input  boolean_output=off  explicit_period=off  period=1  dbl_ovrd=off
  SliceLow : xbsIndex_r3/Slice  mode=Lower Bit Location + Width  nbits=10  bit1=0  base1=MSB of Input  bit0=0  base0=LSB of Input  boolean_output=off  explicit_period=off  period=1  dbl_ovrd=off
  SyncCompare : xbsIndex_r3/Relational  mode=a=b  latency=1  explicit_period=off  period=1  en=off  dbl_ovrd=off  show_param=off
      settings: xl_area=[0, 0, 0, 0, 0, 0, 0]
  SyncConst : xbsIndex_r3/Constant  const=1022  equ=P=C  arith_type=Unsigned  n_bits=10  bin_pt=0  opselect=C  inp2=PCIN>>17  opr=+  inp1=P  carry=CIN  iostate=0  explicit_period=on  period=1  dbl_ovrd=off
  SyncDelay : xbsIndex_r3/Delay  latency=0  reg_retiming=off  explicit_period=off  period=1  en=off  accept_only_valid=off  init_zero=on  dbl_ovrd=off  show_param=off
      settings: xl_area=[0, 0, 0, 0, 0, 0, 0]
  Uncram : Subsystem  AncestorBlock=gavrt_library/uncram  mask(uncram){num_slice=2, slice_width=24, bin_pt=23, arith_type=1}
      mask prompts: num_slice "Number of slices"; slice_width "Slice Width"; bin_pt "Output Binary Point"; arith_type "Output Arithmetic Type (0=Unsigned, 1=Signed, 2=Boolean)"
      mask help: Takes a concatenated input and slices it up into even pieces and reinterprets them as signed fixed point numbers with a given binary point.
      mask init:
      | uncram_init(gcb, ...
      |     'num_slice', num_slice, ...
      |     'slice_width', slice_width, ...
      |     'bin_pt', bin_pt, ...
      |     'arith_type', arith_type);
      settings: AttributesFormatString=Fix_24_23
  ValidCompare : xbsIndex_r3/Relational  mode=a=b  latency=1  explicit_period=off  period=1  en=off  dbl_ovrd=off  show_param=off
      settings: xl_area=[0, 0, 0, 0, 0, 0, 0]
  ValidDelay : xbsIndex_r3/Delay  latency=3  reg_retiming=off  explicit_period=off  period=1  en=off  accept_only_valid=off  init_zero=on  dbl_ovrd=off  show_param=off
      settings: xl_area=[0, 0, 0, 0, 0, 0, 0]
  Zero : xbsIndex_r3/Constant  const=0  equ=P=C  arith_type=Unsigned  n_bits=8  bin_pt=0  opselect=C  inp2=PCIN>>17  opr=+  inp1=P  carry=CIN  iostate=0  explicit_period=on  period=1  dbl_ovrd=off
  vacc_core1 : Subsystem  AncestorBlock=gavrt_library/vacc_core  mask(vacc_core){veclen=1024, arith_type=1, out_bit_width=32, out_bin_pt=23, add_latency=2, bram_latency=2, mux_latency=1}
      mask prompts: veclen "Vector Length"; arith_type "Arithmetic Type (0=Unsigned, 1=Signed)"; out_bit_width "Output Bit Width"; out_bin_pt "Output Binary Point"; add_latency "Add Latency"; bram_latency "BRAM Latency"; mux_latency "Mux Latency"
      mask help:
      | Currently only Signed arithmetic supported
      | acc_en = 0 --> Load a vector (start a new accumulation)
      | acc_en = 1 --> Accumulate
      mask init:
      | vacc_core_init(gcb, ...
      |     'veclen', veclen, ...
      |     'arith_type', arith_type, ...
      |     'out_bit_width', out_bit_width, ...
      |     'out_bin_pt', out_bin_pt, ...
      |     'add_latency', add_latency, ...
      |     'bram_latency', bram_latency, ...
      |     'mux_latency', mux_latency);
  vacc_core2 : Subsystem  AncestorBlock=gavrt_library/vacc_core  mask(vacc_core){veclen=1024, arith_type=1, out_bit_width=32, out_bin_pt=23, add_latency=2, bram_latency=2, mux_latency=1}
      mask prompts: veclen "Vector Length"; arith_type "Arithmetic Type (0=Unsigned, 1=Signed)"; out_bit_width "Output Bit Width"; out_bin_pt "Output Binary Point"; add_latency "Add Latency"; bram_latency "BRAM Latency"; mux_latency "Mux Latency"
      mask help:
      | Currently only Signed arithmetic supported
      | acc_en = 0 --> Load a vector (start a new accumulation)
      | acc_en = 1 --> Accumulate
      mask init: same as dig_int_kurt/vacc/vacc_core1
  valid : Outport
  dout : Outport  Port=2
  wires:
  sync/1 -> SyncDelay/1
  SyncDelay/1 -> OR/1
  [valid] -> AND/1
  AND/1 -> OR/2
  OR/1 -> Counter/1
  Counter/1 -> [count], Slice/1
  [count] -> SliceLow/1
  SliceLow/1 -> SyncCompare/1
  SyncConst/1 -> SyncCompare/2
  SyncCompare/1 -> AND/2
  ValidCompare/1 -> [valid], ValidDelay/1
  acc_len/1 -> ValidCompare/1
  Slice/1 -> ValidCompare/2, AccEnCompare/1
  Zero/1 -> AccEnCompare/2
  ValidDelay/1 -> valid/1
  din/1 -> DinDelay/1
  DinDelay/1 -> Uncram/1(In)
  Cram/1(Out) -> dout/1
  Uncram/1(Out1) -> vacc_core1/1(din)
  AccEnCompare/1 -> vacc_core1/2(acc_en), vacc_core2/2(acc_en)
  vacc_core1/1(dout) -> Cram/1(In1)
  Uncram/2(Out2) -> vacc_core2/1(din)
  vacc_core2/1(dout) -> Cram/2(In2)
